simulink model "DC_SIMC_R2018a"  (R2018a)
settings: Solver=VariableStepAuto  StartTime=0.0  StopTime=2  MaxStep=1e-4  RelTol=1e-3
values from neighbouring files (symbols this model uses):
  b = 20    [DC_SIMC.m]    (also in DC_SIMC_facit.m; DC_parameters.m; DC_parameters_facit.m)
  gr = 200    [DC_SIMC.m]    (also in DC_SIMC_facit.m; DC_parameters.m; DC_parameters_facit.m)
  J = 50*1.5^2    (= 112.5)    [DC_SIMC.m]    (also in DC_SIMC_facit.m; DC_parameters.m; DC_parameters_facit.m)
  k = Vmax / gr / (speed_max*pi/180)    (= 0.954929658551)    [DC_SIMC.m]    (also in DC_SIMC_facit.m; DC_lead_scaling.m = 200; DC_parameters.m; DC_parameters_facit.m)
  k1 = 1/( gr*k + b*R/(gr*k))    (= 0.00522167224505)    [DC_SIMC.m]    (also in DC_SIMC_facit.m; DC_parameters.m; DC_parameters_facit.m)
  Kc = 1/(k1*(tauc+theta))    (= 12452.5884156)    [DC_SIMC_facit.m]
  L = 4e-3    (= 0.004)    [DC_SIMC.m]    (also in DC_SIMC_facit.m; DC_parameters.m; DC_parameters_facit.m)
  R = 5    [DC_SIMC.m]    (also in DC_SIMC_facit.m; DC_parameters.m; DC_parameters_facit.m)
  tauD = tau2    (= 0.0153790942167)    [DC_SIMC_facit.m]
  taudc = J/((gr*k)^2/R + b)    (= 0.0153790942167)    [DC_SIMC.m]    (also in DC_SIMC_facit.m; DC_parameters.m; DC_parameters_facit.m)
  tauI = 4*(tauc + theta)    (= 0.0615163768668)    [DC_SIMC_facit.m]
  Vmax = 400    [DC_SIMC.m]    (also in DC_SIMC_facit.m; DC_parameters.m; DC_parameters_facit.m)
settings Model: Creator=kjartan  LastModifiedBy=kjartan
settings DataIOCC: ReturnWorkspaceOutputs=on
settings DebuggingCC: SFMachineParentedDataDiag=error
settings SFSimCC: SimUseLocalCustomCode=on
settings RTWCC: RTWUseLocalCustomCode=on

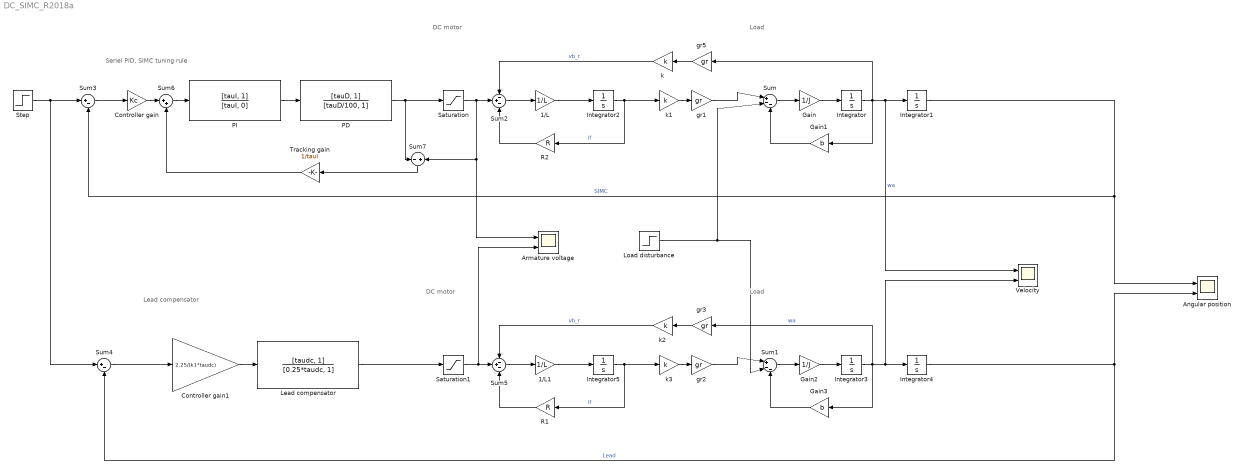
== system DC_SIMC_R2018a ==
  note: Lead compensator
  note: Seriel PID, SIMC tuning rule
  note: Load
  note: DC motor
  note: DC motor
  note: Load
  1/L : Gain  Gain=1/L
  1/L1 : Gain  Gain=1/L
  Angular position : Scope  NumInputPorts=2
  Armature voltage : Scope  NumInputPorts=2
  Controller gain : Gain  Gain=Kc
  Controller gain1 : Gain  Gain=2.25/(k1*taudc)
  Gain : Gain  Gain=1/J
  Gain1 : Gain  Gain=b
  Gain2 : Gain  Gain=1/J
  Gain3 : Gain  Gain=b
  Integrator{,1..5} (6 alike) : Integrator
  Lead compensator : TransferFcn  Numerator=[taudc, 1]  Denominator=[0.25*taudc, 1]
  Load disturbance : Step  After=4000  SampleTime=0
  PD : TransferFcn  Numerator=[tauD, 1]  Denominator=[tauD/100, 1]
  PI : TransferFcn  Numerator=[tauI, 1]  Denominator=[tauI, 0]
  R1 : Gain  Gain=R
  R2 : Gain  Gain=R
  Saturation : Saturate  UpperLimit=Vmax  LowerLimit=-Vmax
  Saturation1 : Saturate  UpperLimit=Vmax  LowerLimit=-Vmax
  Step : Step  Time=0  After=0.1  SampleTime=0
  Sum : Sum  Inputs=|+--
  Sum1 : Sum  Inputs=|+--
  Sum2 : Sum  Inputs=-+-
  Sum3 : Sum  Inputs=|+-
  Sum4 : Sum  Inputs=|+-
  Sum5 : Sum  Inputs=-+-
  Sum6 : Sum  Inputs=|++
  Sum7 : Sum  Inputs=-|+
  Tracking gain : Gain  Gain=1/tauI
  Velocity : Scope  NumInputPorts=2
  gr{1..3,5} (4 alike) : Gain  Gain=gr
  k{,1..3} (4 alike) : Gain  Gain=k
  wires:
  gr5/1 -> k/1
  R2/1 -> Sum2/3
  Integrator2/1 -> R2/1, k1/1  "if"
  Sum2/1 -> 1/L/1
  k1/1 -> gr1/1
  1/L/1 -> Integrator2/1
  k/1 -> Sum2/1  "vb_r"
  gr1/1 -> Sum/1
  Gain/1 -> Integrator/1
  Integrator/1 -> Gain1/1, gr5/1, Velocity/1, Integrator1/1  "wa"
  Integrator1/1 -> Angular position/1, Sum3/2  "SIMC"
  Controller gain/1 -> Sum6/1
  Sum3/1 -> Controller gain/1
  Step/1 -> Sum4/1, Sum3/1
  PD/1 -> Sum7/1, Saturation/1
  Sum/1 -> Gain/1
  Gain1/1 -> Sum/3
  PI/1 -> PD/1
  Sum4/1 -> Controller gain1/1
  Integrator5/1 -> R1/1, k3/1  "if"
  Lead compensator/1 -> Saturation1/1
  Gain2/1 -> Integrator3/1
  Integrator4/1 -> Sum4/2, Angular position/2  "Lead"
  Sum5/1 -> 1/L1/1
  Load disturbance/1 -> Sum1/2, Sum/2
  k3/1 -> gr2/1
  gr2/1 -> Sum1/1
  Gain3/1 -> Sum1/3
  1/L1/1 -> Integrator5/1
  R1/1 -> Sum5/3
  gr3/1 -> k2/1
  k2/1 -> Sum5/1  "vb_r"
  Integrator3/1 -> Gain3/1, gr3/1, Velocity/2, Integrator4/1  "wa"
  Sum1/1 -> Gain2/1
  Controller gain1/1 -> Lead compensator/1
  Saturation/1 -> Armature voltage/1, Sum7/2, Sum2/2
  Saturation1/1 -> Armature voltage/2, Sum5/2
  Sum6/1 -> PI/1
  Sum7/1 -> Tracking gain/1
  Tracking gain/1 -> Sum6/2
